simulink model "Copy_of_mpcACCWithSensorFusion"  (R2023b)
settings: Solver=FixedStepAuto  StartTime=0.0  StopTime=34  FixedStep=0.1  RelTol=1e-3
values from neighbouring files (symbols this model uses):
  pfcsubsystem_data =     [pfc_controller_data.mat]    (also in pfc_data.mat; pfc_subsystem_data.mat)
  posSelector = [1,0,0,0,0,0; 0,0,1,0,0,0]    [setUpACCWorkspaceVars.m]
  Ts = 0.1    [mainACCcode.m]    (also in setUpACCWorkspaceVars.m)
undefined symbols (not defined in the file or in its folder): hasLag, InitialLongVel, NumEgoStates, PredictionHorizon
libraries: mpcsigdimcheck_private x19, simulink x2, mpclib x2, trackingutilitieslib x1, drivinglib x1
(part 1 of 2)
settings Model: Creator=The MathWorks, Inc.  LastModifiedBy=Subhadeep Das
settings SolverCC: AlgebraicLoopSolver=TrustRegion  MinimalZcImpactIntegration=on
settings DataIOCC: SaveOutput=off  SignalLogging=off  SaveTime=off  ReturnWorkspaceOutputs=off
settings OptimizationCC: DefaultParameterBehavior=Inlined  InlineInvariantSignals=on  PassReuseOutputArgsAs=Individual arguments  ZeroExternalMemoryAtStartup=off  ZeroInternalMemoryAtStartup=off  OptimizeBlockOrder=speed  EfficientTunableParamExpr=on
settings DebuggingCC: ParameterTunabilityLossMsg=error  UnconnectedInputMsg=warning  UnconnectedOutputMsg=warning  UnconnectedLineMsg=warning  ArithmeticOperatorsInVariantConditions=warning
settings HardwareCC: ProdLongLongMode=on
settings ModelReferenceCC: EnableRefExpFcnMdlSchedulingChecks=on  PropagateVarSize=Only when enabling
settings SFSimCC: SimUseLocalCustomCode=off  MATLABDynamicMemAlloc=off  CustomCodeUndefinedFunction=UseInterfaceOnly  SimTargetLang=C++
settings RTWCC: Description=Embedded Coder  SystemTargetFile=ert.tlc  TemplateMakefile=ert_default_tmf  GenerateReport=on  RTWUseLocalCustomCode=off  BuildConfiguration=Faster Runs  IncludeHyperlinkInReport=on  LaunchReport=on  TargetLang=C++  GenerateTraceInfo=on  GenerateTraceReport=on  GenerateTraceReportSl=on  GenerateTraceReportSf=on  GenerateTraceReportEml=on  GenerateCodeMetricsReport=on  DLArmComputeVersion=19.05
settings CodeAppCC: ForceParamTrailComments=on  IgnoreCustomStorageClasses=off  MaxIdLength=63  OperatorAnnotations=on  SimulinkDataObjDesc=on  SFDataObjDesc=on  CustomSymbolStrFcn=$N$M$F  InsertBlockDesc=on
settings ERTTargetCC: TargetLangStandard=C++03 (ISO)  GenerateSampleERTMain=on  CombineSignalStateStructs=on  SuppressErrorStatus=on  CodeInterfacePackaging=C++ class  InlinedParameterPlacement=NonHierarchical  RootIOFormat=Structure reference  RTWCAPISignals=on  ERTCustomFileTemplate=example_file_process.tlc

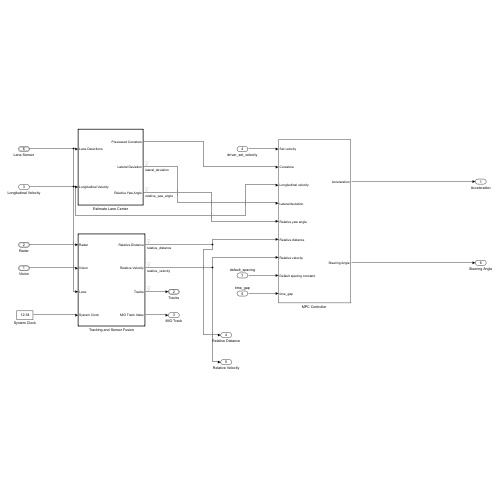
[thumbnail: Simulink's stored preview of the top-level diagram]
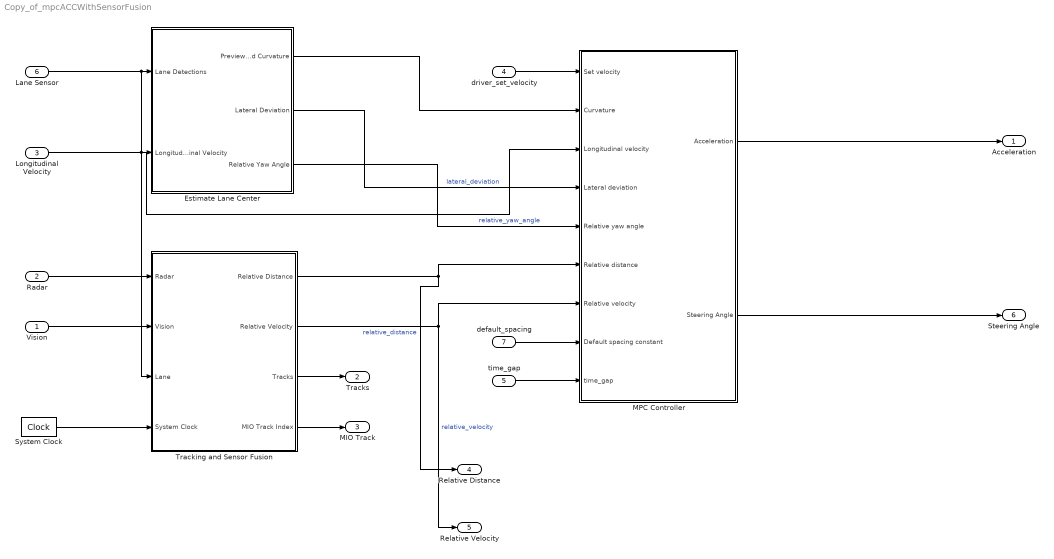
== system Copy_of_mpcACCWithSensorFusion ==
  Vision : Inport  OutDataTypeStr=Bus: BusVision  PortDimensions=[1 1]  SampleTime=[0.10000000000000001,0]  BusOutputAsStruct=on
  Radar : Inport  Port=2  OutDataTypeStr=Bus: BusRadar  PortDimensions=[1 1]  SampleTime=[0.10000000000000001,0]  BusOutputAsStruct=on
  Longitudinal Velocity : Inport  Port=3  OutDataTypeStr=double  PortDimensions=1  SampleTime=[0.10000000000000001,0]
  driver_set_velocity : Inport  Port=4
  time_gap : Inport  Port=5
  Lane Sensor : Inport  Port=6  OutDataTypeStr=Bus: LaneSensor
  default_spacing : Inport  Port=7
  Estimate Lane Center : Subsystem  TreatAsAtomicUnit=on  VariantControl=v2
      settings: RTWFileNameOpts=Use function name
  "MPC Controller " : Subsystem
  System Clock : DigitalClock  SampleTime=Ts
  Tracking and Sensor Fusion : Subsystem  TreatAsAtomicUnit=on
      settings: RTWFileNameOpts=Use function name
  "Acceleration " : Outport  OutDataTypeStr=double  PortDimensions=1  SampleTime=[0.10000000000000001,0]  VectorParamsAs1DForOutWhenUnconnected=off
  Tracks : Outport  Port=2  OutDataTypeStr=Bus:BusMultiObjectTracker1  PortDimensions=[1 1]  SampleTime=[0.10000000000000001,0]  VectorParamsAs1DForOutWhenUnconnected=off  BusOutputAsStruct=on
  MIO Track : Outport  Port=3  OutDataTypeStr=double  PortDimensions=1  SampleTime=[0.10000000000000001,0]  VectorParamsAs1DForOutWhenUnconnected=off  BusOutputAsStruct=on
  Relative Distance : Outport  Port=4
  Relative Velocity : Outport  Port=5
  Steering Angle : Outport  Port=6
  wires:
  Tracking and Sensor Fusion/3(Tracks) -> Tracks/1
  Vision/1 -> Tracking and Sensor Fusion/2(Vision)
  Radar/1 -> Tracking and Sensor Fusion/1(Radar)
  Tracking and Sensor Fusion/4(MIO Track Index) -> MIO Track/1
  Longitudinal Velocity/1 -> "MPC Controller "/3(Longitudinal velocity), Estimate Lane Center/2(Longitudinal Velocity)
  Lane Sensor/1 -> Tracking and Sensor Fusion/3(Lane), Estimate Lane Center/1(Lane Detections)
  System Clock/1 -> Tracking and Sensor Fusion/4(System Clock)
  Tracking and Sensor Fusion/1(Relative Distance) -> Relative Distance/1, "MPC Controller "/6(Relative distance)  "relative_distance"
  Tracking and Sensor Fusion/2(Relative Velocity) -> Relative Velocity/1, "MPC Controller "/7(Relative velocity)  "relative_velocity"
  driver_set_velocity/1 -> "MPC Controller "/1(Set velocity)
  time_gap/1 -> "MPC Controller "/9(time_gap)
  Estimate Lane Center/3(Relative Yaw Angle) -> "MPC Controller "/5(Relative yaw angle)  "relative_yaw_angle"
  Estimate Lane Center/2(Lateral Deviation) -> "MPC Controller "/4(Lateral deviation)  "lateral_deviation"
  Estimate Lane Center/1(Previewed Curvature) -> "MPC Controller "/2(Curvature)
  default_spacing/1 -> "MPC Controller "/8(Default spacing constant)
  "MPC Controller "/1(Acceleration) -> "Acceleration "/1
  "MPC Controller "/2(Steering Angle) -> Steering Angle/1

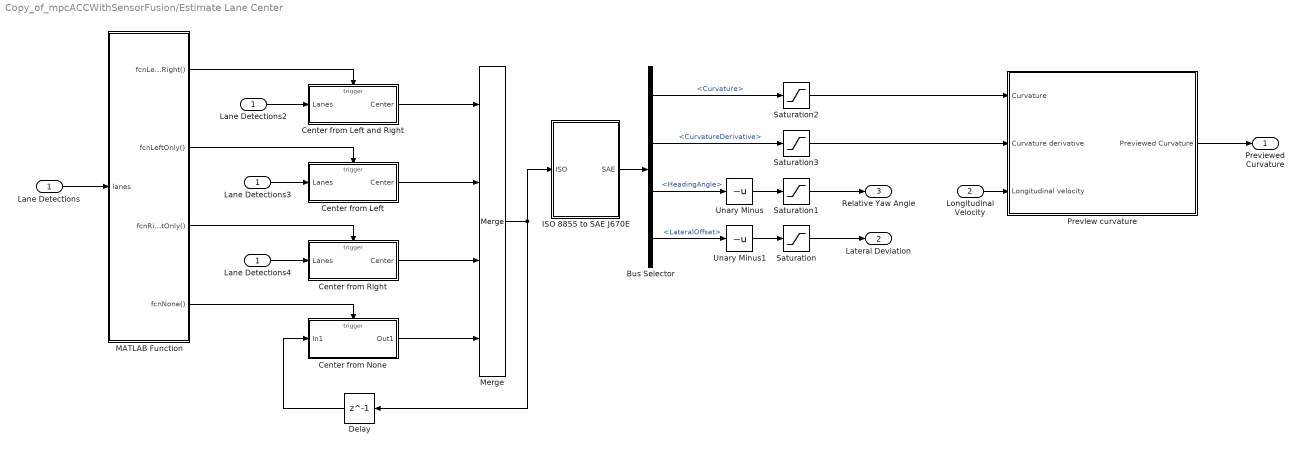
== system Copy_of_mpcACCWithSensorFusion/Estimate Lane Center ==
  Lane Detections : Inport
  Longitudinal Velocity : Inport  Port=2
  Bus Selector : BusSelector  OutputSignals=Curvature,CurvatureDerivative,HeadingAngle,LateralOffset
  Center from Left : Subsystem  TreatAsAtomicUnit=on
  Center from Left and Right : Subsystem  TreatAsAtomicUnit=on
  Center from None : Subsystem  TreatAsAtomicUnit=on
  Center from Right : Subsystem  TreatAsAtomicUnit=on
  Delay : Delay  DelayLength=1
  ISO 8855 to SAE J670E : Subsystem
  Lane Detections2 : InportShadow
  Lane Detections3 : InportShadow
  Lane Detections4 : InportShadow
  MATLAB Function : MATLAB Function  TreatAsAtomicUnit=on
  Merge : Merge  Inputs=4
  Preview curvature : Subsystem
  Saturation : Saturate
  Saturation1 : Saturate  UpperLimit=0.6  LowerLimit=-0.6
  Saturation2 : Saturate  UpperLimit=0.15  LowerLimit=-0.15
  Saturation3 : Saturate  UpperLimit=0.06  LowerLimit=-0.06
  Unary Minus : UnaryMinus
  Unary Minus1 : UnaryMinus
  Previewed Curvature : Outport  VectorParamsAs1DForOutWhenUnconnected=off
  Lateral Deviation : Outport  Port=2  VectorParamsAs1DForOutWhenUnconnected=off
  Relative Yaw Angle : Outport  Port=3  VectorParamsAs1DForOutWhenUnconnected=off
  wires:
  Center from Right/1(Center) -> Merge/3
  Lane Detections3/1 -> Center from Left/1(Lanes)
  Lane Detections4/1 -> Center from Right/1(Lanes)
  MATLAB Function/2(fcnLeftOnly()) -> Center from Left/Trigger
  Center from None/1(Out1) -> Merge/4
  MATLAB Function/1(fcnLeftAndRight()) -> Center from Left and Right/Trigger
  Delay/1 -> Center from None/1(In1)
  Center from Left and Right/1(Center) -> Merge/1
  Lane Detections/1 -> MATLAB Function/1(lanes)
  Lane Detections2/1 -> Center from Left and Right/1(Lanes)
  MATLAB Function/3(fcnRightOnly()) -> Center from Right/Trigger
  MATLAB Function/4(fcnNone()) -> Center from None/Trigger
  Center from Left/1(Center) -> Merge/2
  Merge/1 -> ISO 8855 to SAE J670E/1(ISO), Delay/1
  Saturation3/1 -> Preview curvature/2(Curvature derivative)
  Saturation2/1 -> Preview curvature/1(Curvature)
  Saturation1/1 -> Relative Yaw Angle/1
  Saturation/1 -> Lateral Deviation/1
  Unary Minus/1 -> Saturation1/1
  Preview curvature/1(Previewed Curvature) -> Previewed Curvature/1
  Longitudinal Velocity/1 -> Preview curvature/3(Longitudinal velocity)
  Bus Selector/2 -> Saturation3/1  "<CurvatureDerivative>"
  Bus Selector/1 -> Saturation2/1  "<Curvature>"
  Unary Minus1/1 -> Saturation/1
  Bus Selector/4 -> Unary Minus1/1  "<LateralOffset>"
  Bus Selector/3 -> Unary Minus/1  "<HeadingAngle>"
  ISO 8855 to SAE J670E/1(SAE) -> Bus Selector/1

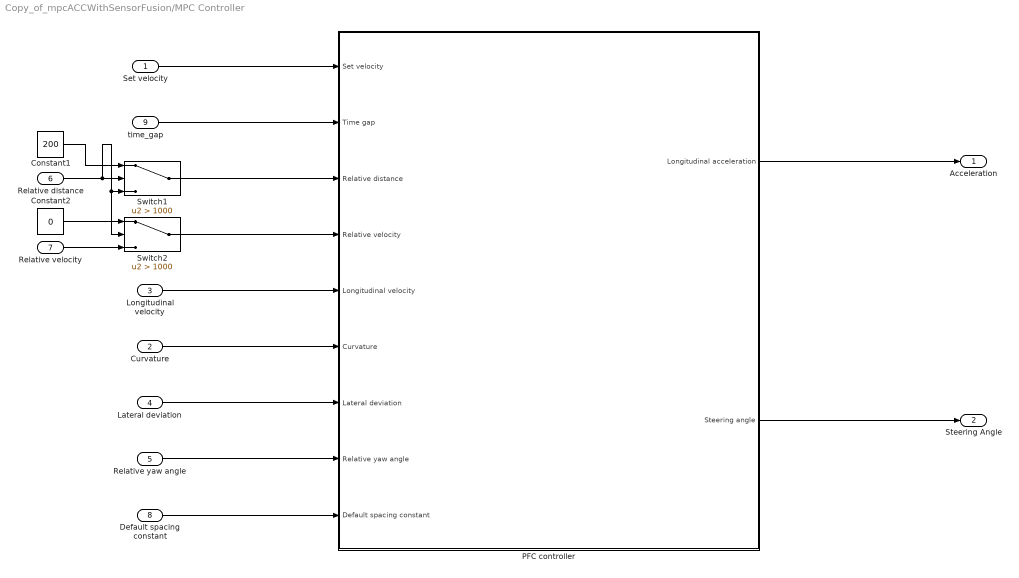
== system Copy_of_mpcACCWithSensorFusion/MPC Controller  ==
  Set velocity : Inport
  Curvature : Inport  Port=2
  Longitudinal velocity : Inport  Port=3
  Lateral deviation : Inport  Port=4
  Relative yaw angle : Inport  Port=5
  Relative distance : Inport  Port=6
  Relative velocity : Inport  Port=7
  Default spacing constant : Inport  Port=8
  time_gap : Inport  Port=9
  Constant1 : Constant  Value=200
  Constant2 : Constant  Value=0
  PFC controller : Subsystem  TreatAsAtomicUnit=on  VariantControl=Variant2
      settings: LibrarySourceBlock=mpcadaslib/Path Following Control System  RTWFileNameOpts=Use function name
  Switch1 : Switch  Criteria=u2 > Threshold  Threshold=1000  SaturateOnIntegerOverflow=off  InputSameDT=off
  Switch2 : Switch  Criteria=u2 > Threshold  Threshold=1000  SaturateOnIntegerOverflow=off  InputSameDT=off
  Acceleration : Outport  VectorParamsAs1DForOutWhenUnconnected=off
  Steering Angle : Outport  Port=2  VectorParamsAs1DForOutWhenUnconnected=off
  wires:
  PFC controller/1(Longitudinal acceleration) -> Acceleration/1
  PFC controller/2(Steering angle) -> Steering Angle/1
  Set velocity/1 -> PFC controller/1(Set velocity)
  time_gap/1 -> PFC controller/2(Time gap)
  Relative distance/1 -> Switch2/2, Switch1/3, Switch1/2
  Constant1/1 -> Switch1/1
  Switch1/1 -> PFC controller/3(Relative distance)
  Relative velocity/1 -> Switch2/3
  Constant2/1 -> Switch2/1
  Switch2/1 -> PFC controller/4(Relative velocity)
  Longitudinal velocity/1 -> PFC controller/5(Longitudinal velocity)
  Curvature/1 -> PFC controller/6(Curvature)
  Lateral deviation/1 -> PFC controller/7(Lateral deviation)
  Relative yaw angle/1 -> PFC controller/8(Relative yaw angle)
  Default spacing constant/1 -> PFC controller/9(Default spacing constant)

== system Copy_of_mpcACCWithSensorFusion/Tracking and Sensor Fusion ==
  note: Sensor Fusion
  Radar : Inport  OutDataTypeStr=Bus: BusRadar  PortDimensions=[1 1]  BusOutputAsStruct=on
  Vision : Inport  Port=2  OutDataTypeStr=Bus: BusVision  PortDimensions=[1 1]  BusOutputAsStruct=on
  Lane : Inport  Port=3  OutDataTypeStr=Bus: LaneSensor  BusOutputAsStruct=on
  System Clock : Inport  Port=4  OutDataTypeStr=double  PortDimensions=[1 1]
  Detection Concatenation1 : trackingutilitieslib/Detection Concatenation  NumInputs=2  BusNameSource=Auto  BusName=BusDetectionConcatenation1  SimulateUsing=Interpreted execution
  Find Lead Car : MATLAB Function  TreatAsAtomicUnit=on
  Multi-Object Tracker : drivinglib/Multi-Object Tracker  TrackerIndex=uint32( 0 )  FilterInitializationFcn=initcvekf  AssignmentThreshold=assigThresh  ConfirmationThreshold=[ 2, 3 ]  DeletionThreshold=[ 5, 5 ]  MaxNumTracks=numTracks  MaxNumSensors=numSensors  OOSMHandling=Terminate  StateParametersSimulink=struct  HasStateParametersInput=off  TimeInputSource=Input port  HasCostMatrixInput=off  HasDetectableTrackIDsInput=off  BusNameSource=Property  BusName=BusMultiObjectTracker1  TentativeTracksOutputPort=off  AllTracksOutputPort=off  SimulateUsing=Interpreted execution
  Position Selector : Constant  Value=posSelector
  Relative Distance : Outport  VectorParamsAs1DForOutWhenUnconnected=off
  Relative Velocity : Outport  Port=2  VectorParamsAs1DForOutWhenUnconnected=off
  Tracks : Outport  Port=3  OutDataTypeStr=Bus:BusMultiObjectTracker1  PortDimensions=[1 1]  VectorParamsAs1DForOutWhenUnconnected=off  BusOutputAsStruct=on
  MIO Track Index : Outport  Port=4  VectorParamsAs1DForOutWhenUnconnected=off
  wires:
  Find Lead Car/2(vx) -> Relative Velocity/1
  Find Lead Car/3(mioTrackIndex) -> MIO Track Index/1
  Find Lead Car/1(x) -> Relative Distance/1
  Position Selector/1 -> Find Lead Car/3(positionSelector)
  Lane/1 -> Find Lead Car/2(lane)
  Detection Concatenation1/1 -> Multi-Object Tracker/1
  Multi-Object Tracker/1 -> Find Lead Car/1(confirmedTracks), Tracks/1
  System Clock/1 -> Multi-Object Tracker/2
  Vision/1 -> Detection Concatenation1/1
  Radar/1 -> Detection Concatenation1/2

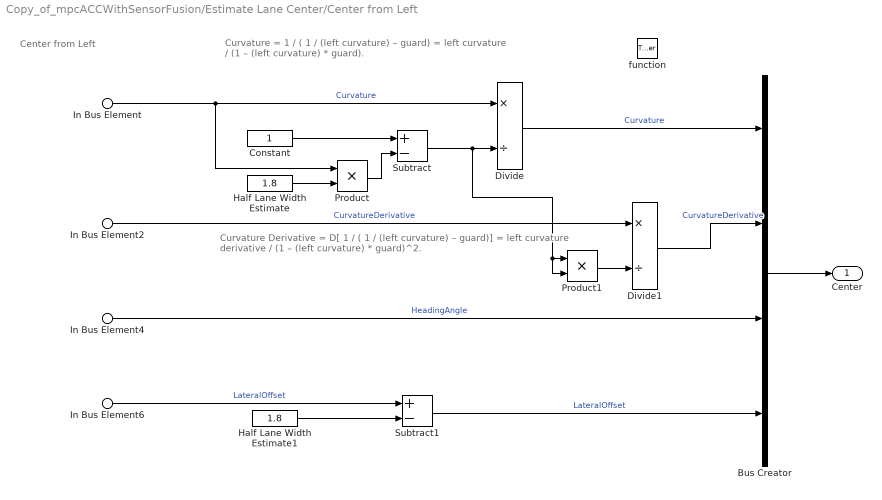
== system Copy_of_mpcACCWithSensorFusion/Estimate Lane Center/Center from Left ==
  note: Curvature Derivative
      | = D[ 1 / ( 1 / (left curvature) – guard)]
      | = left curvature derivative / (1 – (left curvature) * guard)^2.
  note: Center from Left
  note: Curvature
      | = 1 / ( 1 / (left curvature) – guard)
      | = left curvature / (1 – (left curvature) * guard).
  In Bus Element : Inport  PortName=Lanes  Element=Left.Curvature
  In Bus Element2 : Inport  PortName=Lanes  Element=Left.CurvatureDerivative
  In Bus Element4 : Inport  PortName=Lanes  Element=Left.HeadingAngle
  In Bus Element6 : Inport  PortName=Lanes  Element=Left.LateralOffset
  function : TriggerPort  TriggerType=function-call  VariantControl=Variant
  Bus Creator : BusCreator  Inputs=4
  Constant : Constant  OutDataTypeStr=Inherit: Inherit via back propagation
  Divide : Product  Inputs=*/
  Divide1 : Product  Inputs=*/
  Half Lane Width Estimate : Constant  Value=1.8  OutDataTypeStr=Inherit: Inherit via back propagation
  Half Lane Width Estimate1 : Constant  Value=1.8  OutDataTypeStr=Inherit: Inherit via back propagation
  Product : Product
  Product1 : Product
  Subtract : Sum  Inputs=+-
  Subtract1 : Sum  Inputs=+-
  Center : Outport  VectorParamsAs1DForOutWhenUnconnected=off
  wires:
  Product/1 -> Subtract/2
  Half Lane Width Estimate1/1 -> Subtract1/2
  In Bus Element6/1 -> Subtract1/1  "LateralOffset"
  Product1/1 -> Divide1/2
  In Bus Element2/1 -> Divide1/1  "CurvatureDerivative"
  Constant/1 -> Subtract/1
  Half Lane Width Estimate/1 -> Product/2
  Subtract/1 -> Divide/2, Product1/1, Product1/2
  In Bus Element/1 -> Divide/1, Product/1  "Curvature"
  Subtract1/1 -> Bus Creator/4  "LateralOffset"
  In Bus Element4/1 -> Bus Creator/3  "HeadingAngle"
  Divide/1 -> Bus Creator/1  "Curvature"
  Divide1/1 -> Bus Creator/2  "CurvatureDerivative"
  Bus Creator/1 -> Center/1

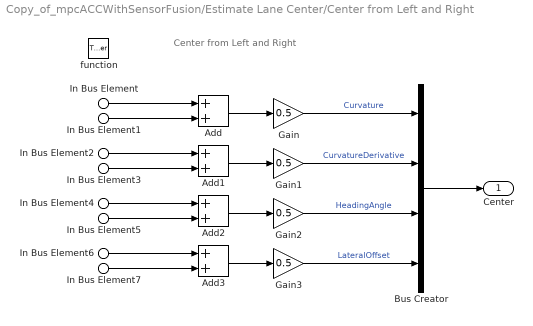
== system Copy_of_mpcACCWithSensorFusion/Estimate Lane Center/Center from Left and Right ==
  note: Center from Left and Right
  In Bus Element : Inport  PortName=Lanes  Element=Left.Curvature
  In Bus Element2 : Inport  PortName=Lanes  Element=Left.CurvatureDerivative
  In Bus Element4 : Inport  PortName=Lanes  Element=Left.HeadingAngle
  In Bus Element6 : Inport  PortName=Lanes  Element=Left.LateralOffset
  In Bus Element1 : Inport  PortName=Lanes  Element=Right.Curvature
  In Bus Element3 : Inport  PortName=Lanes  Element=Right.CurvatureDerivative
  In Bus Element5 : Inport  PortName=Lanes  Element=Right.HeadingAngle
  In Bus Element7 : Inport  PortName=Lanes  Element=Right.LateralOffset
  function : TriggerPort  TriggerType=function-call  VariantControl=Variant
  Add{,1..3} (4 alike) : Sum
  Bus Creator : BusCreator  Inputs=4
  Gain{,1..3} (4 alike) : Gain  Gain=0.5
  Center : Outport  VectorParamsAs1DForOutWhenUnconnected=off
  wires:
  In Bus Element6/1 -> Add3/1
  In Bus Element7/1 -> Add3/2
  In Bus Element5/1 -> Add2/2
  In Bus Element4/1 -> Add2/1
  In Bus Element3/1 -> Add1/2
  In Bus Element2/1 -> Add1/1
  In Bus Element1/1 -> Add/2
  In Bus Element/1 -> Add/1
  Bus Creator/1 -> Center/1
  Gain3/1 -> Bus Creator/4  "LateralOffset"
  Add3/1 -> Gain3/1
  Gain2/1 -> Bus Creator/3  "HeadingAngle"
  Add2/1 -> Gain2/1
  Gain1/1 -> Bus Creator/2  "CurvatureDerivative"
  Add1/1 -> Gain1/1
  Gain/1 -> Bus Creator/1  "Curvature"
  Add/1 -> Gain/1

== system Copy_of_mpcACCWithSensorFusion/Estimate Lane Center/Center from None ==
  In1 : Inport
  function : TriggerPort  TriggerType=function-call  VariantControl=Variant
  Out1 : Outport  VectorParamsAs1DForOutWhenUnconnected=off
  wires:
  In1/1 -> Out1/1

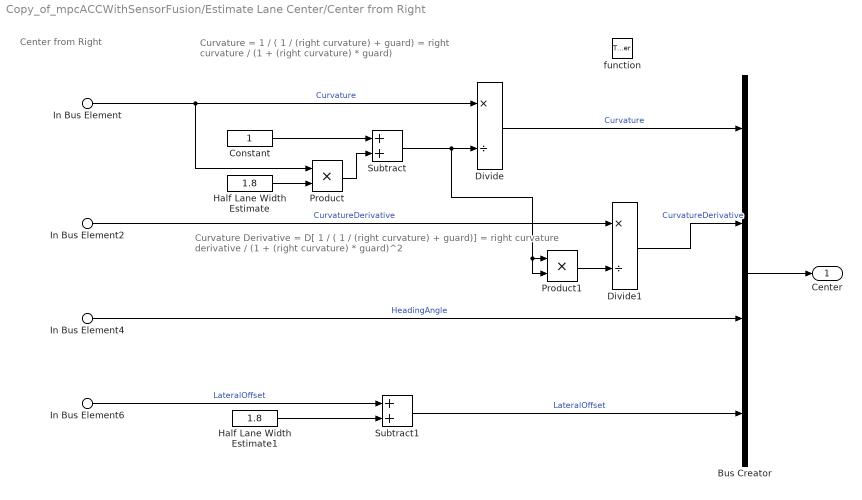
== system Copy_of_mpcACCWithSensorFusion/Estimate Lane Center/Center from Right ==
  note: Curvature Derivative
      | = D[ 1 / ( 1 / (right curvature) + guard)]
      | = right curvature derivative / (1 + (right curvature) * guard)^2
  note: Curvature
      | = 1 / ( 1 / (right curvature) + guard)
      | = right curvature / (1 + (right curvature) * guard)
  note: Center from Right
  In Bus Element : Inport  PortName=Lanes  Element=Right.Curvature
  In Bus Element2 : Inport  PortName=Lanes  Element=Right.CurvatureDerivative
  In Bus Element4 : Inport  PortName=Lanes  Element=Right.HeadingAngle
  In Bus Element6 : Inport  PortName=Lanes  Element=Right.LateralOffset
  function : TriggerPort  TriggerType=function-call  VariantControl=Variant
  Bus Creator : BusCreator  Inputs=4
  Constant : Constant  OutDataTypeStr=Inherit: Inherit via back propagation
  Divide : Product  Inputs=*/
  Divide1 : Product  Inputs=*/
  Half Lane Width Estimate : Constant  Value=1.8  OutDataTypeStr=Inherit: Inherit via back propagation
  Half Lane Width Estimate1 : Constant  Value=1.8  OutDataTypeStr=Inherit: Inherit via back propagation
  Product : Product
  Product1 : Product
  Subtract : Sum
  Subtract1 : Sum
  Center : Outport  VectorParamsAs1DForOutWhenUnconnected=off
  wires:
  Half Lane Width Estimate/1 -> Product/2
  Product/1 -> Subtract/2
  Constant/1 -> Subtract/1
  Subtract/1 -> Divide/2, Product1/1, Product1/2
  In Bus Element/1 -> Divide/1, Product/1  "Curvature"
  Bus Creator/1 -> Center/1
  Subtract1/1 -> Bus Creator/4  "LateralOffset"
  Divide/1 -> Bus Creator/1  "Curvature"
  In Bus Element6/1 -> Subtract1/1  "LateralOffset"
  Half Lane Width Estimate1/1 -> Subtract1/2
  In Bus Element4/1 -> Bus Creator/3  "HeadingAngle"
  Product1/1 -> Divide1/2
  Divide1/1 -> Bus Creator/2  "CurvatureDerivative"
  In Bus Element2/1 -> Divide1/1  "CurvatureDerivative"

== system Copy_of_mpcACCWithSensorFusion/Estimate Lane Center/ISO 8855 to SAE J670E ==
  ISO : Inport
  Bus Creator : BusCreator  Inputs=4
  Bus Selector : BusSelector  OutputSignals=CurvatureDerivative,Curvature,HeadingAngle,LateralOffset
  Signal Specification : SignalSpecification  Unit=1/m^2
  Signal Specification1 : SignalSpecification  Unit=1/m
  Signal Specification2 : SignalSpecification  Unit=rad
  Signal Specification3 : SignalSpecification  Unit=m
  Unary Minus{,1..3} (4 alike) : UnaryMinus
  SAE : Outport  VectorParamsAs1DForOutWhenUnconnected=off
  wires:
  ISO/1 -> Bus Selector/1
  Bus Selector/2 -> Unary Minus/1  "<Curvature>"
  Bus Selector/1 -> Unary Minus1/1  "<CurvatureDerivative>"
  Bus Selector/3 -> Unary Minus2/1  "<HeadingAngle>"
  Bus Selector/4 -> Unary Minus3/1  "<LateralOffset>"
  Bus Creator/1 -> SAE/1
  Signal Specification/1 -> Bus Creator/2  "Curvature"
  Unary Minus1/1 -> Signal Specification1/1
  Unary Minus2/1 -> Signal Specification2/1
  Unary Minus3/1 -> Signal Specification3/1
  Unary Minus/1 -> Signal Specification/1
  Signal Specification1/1 -> Bus Creator/1  "CurvatureDerivative"
  Signal Specification2/1 -> Bus Creator/3  "HeadingAngle"
  Signal Specification3/1 -> Bus Creator/4  "LateralOffset"

== system Copy_of_mpcACCWithSensorFusion/Estimate Lane Center/Preview curvature ==
  Curvature : Inport
  Curvature derivative : Inport  Port=2
  Longitudinal velocity : Inport  Port=3
  Gain : Gain  Gain=[0:Ts:PredictionHorizon*Ts]'
  Product : Product
  Sum : Sum
  Previewed Curvature : Outport  VectorParamsAs1DForOutWhenUnconnected=off
  wires:
  Sum/1 -> Previewed Curvature/1
  Curvature/1 -> Sum/1
  Gain/1 -> Sum/2
  Product/1 -> Gain/1
  Longitudinal velocity/1 -> Product/2
  Curvature derivative/1 -> Product/1

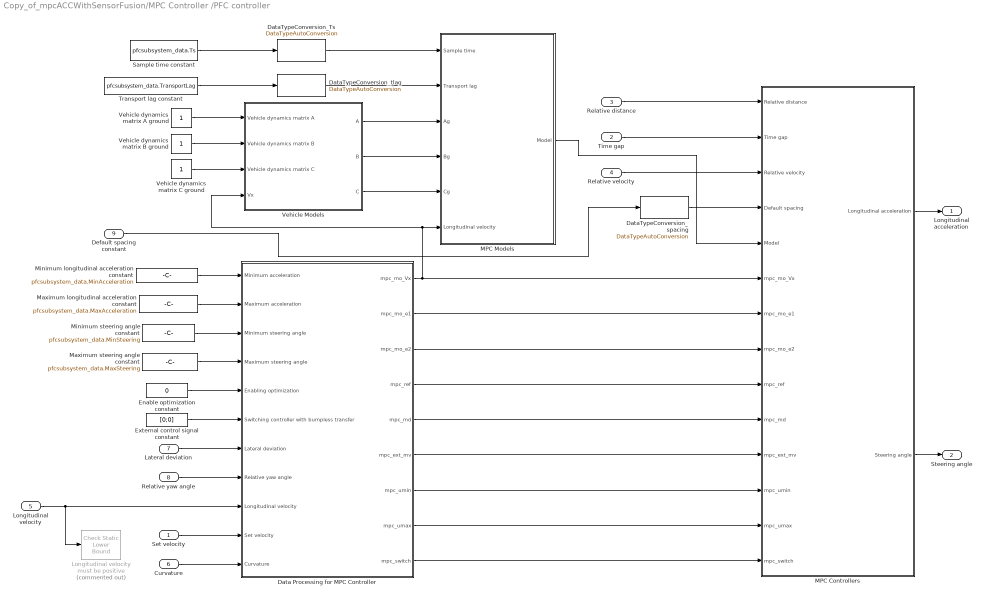
== system Copy_of_mpcACCWithSensorFusion/MPC Controller /PFC controller ==
  Set velocity : Inport
  Time gap : Inport  Port=2
  Relative distance : Inport  Port=3
  Relative velocity : Inport  Port=4
  Longitudinal velocity : Inport  Port=5
  Curvature : Inport  Port=6
  Lateral deviation : Inport  Port=7
  Relative yaw angle : Inport  Port=8
  Default spacing constant : Inport  Port=9
  Data Processing for MPC Controller : Subsystem
  DataTypeConversion_Ts : mpcsigdimcheck_private/DataTypeAutoConversion  datatypestr=pfcsubsystem_data.DataType
  DataTypeConversion_spacing : mpcsigdimcheck_private/DataTypeAutoConversion  datatypestr=pfcsubsystem_data.DataType
  DataTypeConversion_tlag : mpcsigdimcheck_private/DataTypeAutoConversion  datatypestr=pfcsubsystem_data.DataType
  Enable optimization constant : Constant  Value=0  OutDataTypeStr=pfcsubsystem_data.DataType
  External control signal constant : Constant  Value=[0;0]  VectorParams1D=off  OutDataTypeStr=pfcsubsystem_data.DataType
  Longitudinal velocity must be positive : simulink/Model Verification/Check Static  Lower Bound  Description=0 < u  Commented=on  min=0  min_included=off  enabled=on  stopWhenAssertionFail=on  export=off  icon=graphic
  MPC Controllers : Subsystem  Variant=on  VariantControlMode=label  VariantControl=Variant1  LabelModeActiveChoice=pathFollowingHasSpacingCtrl
  MPC Models : Subsystem  Variant=on  VariantControlMode=label  VariantControl=Variant1  LabelModeActiveChoice=pathFollowingHasSpacingCtrl
  Maximum longitudinal acceleration constant : Constant  Value=pfcsubsystem_data.MaxAcceleration  OutDataTypeStr=pfcsubsystem_data.DataType
  Maximum steering angle constant : Constant  Value=pfcsubsystem_data.MaxSteering  OutDataTypeStr=pfcsubsystem_data.DataType
  Minimum longitudinal acceleration constant : Constant  Value=pfcsubsystem_data.MinAcceleration  OutDataTypeStr=pfcsubsystem_data.DataType
  Minimum steering angle constant : Constant  Value=pfcsubsystem_data.MinSteering  OutDataTypeStr=pfcsubsystem_data.DataType
  Sample time constant : Constant  Value=pfcsubsystem_data.Ts  OutDataTypeStr=pfcsubsystem_data.DataType
  Transport lag constant : Constant  Value=pfcsubsystem_data.TransportLag  OutDataTypeStr=pfcsubsystem_data.DataType
  Vehicle Models : Subsystem  Variant=on  VariantControlMode=label  VariantControl=Variant1  LabelModeActiveChoice=useVehicleParameters
  Vehicle dynamics matrix A ground : Constant  OutDataTypeStr=pfcsubsystem_data.DataType
  Vehicle dynamics matrix B ground : Constant  OutDataTypeStr=pfcsubsystem_data.DataType
  Vehicle dynamics matrix C ground : Constant  OutDataTypeStr=pfcsubsystem_data.DataType
  Longitudinal acceleration : Outport  PortDimensions=1  VectorParamsAs1DForOutWhenUnconnected=off
  Steering angle : Outport  Port=2  VectorParamsAs1DForOutWhenUnconnected=off
  wires:
  MPC Controllers/1(" Longitudinal acceleration") -> Longitudinal acceleration/1
  Default spacing constant/1 -> DataTypeConversion_spacing/1
  Data Processing for MPC Controller/9(mpc_switch) -> MPC Controllers/14("mpc_switch ")
  MPC Models/1(" Model") -> MPC Controllers/5("Model ")
  Data Processing for MPC Controller/8(mpc_umax) -> MPC Controllers/13("mpc_umax ")
  MPC Controllers/2("  Steering angle") -> Steering angle/1
  Data Processing for MPC Controller/1(mpc_mo_Vx) -> MPC Models/6("Longitudinal velocity "), Vehicle Models/4("Vx "), MPC Controllers/6("mpc_mo_Vx ")
  Data Processing for MPC Controller/5(mpc_md) -> MPC Controllers/10("mpc_md ")
  Data Processing for MPC Controller/3(mpc_mo_e2) -> MPC Controllers/8("mpc_mo_e2 ")
  Data Processing for MPC Controller/4(mpc_ref) -> MPC Controllers/9("mpc_ref ")
  Longitudinal velocity/1 -> Longitudinal velocity must be positive/1, Data Processing for MPC Controller/9(Longitudinal velocity)
  Data Processing for MPC Controller/2(mpc_mo_e1) -> MPC Controllers/7("mpc_mo_e1 ")
  Data Processing for MPC Controller/6(mpc_ext_mv) -> MPC Controllers/11("mpc_ext_mv ")
  Data Processing for MPC Controller/7(mpc_umin) -> MPC Controllers/12("mpc_umin ")
  Curvature/1 -> Data Processing for MPC Controller/11(Curvature)
  Set velocity/1 -> Data Processing for MPC Controller/10(Set velocity)
  Lateral deviation/1 -> Data Processing for MPC Controller/7(Lateral deviation)
  Relative yaw angle/1 -> Data Processing for MPC Controller/8(Relative yaw angle)
  Maximum longitudinal acceleration constant/1 -> Data Processing for MPC Controller/2(Maximum acceleration)
  Maximum steering angle constant/1 -> Data Processing for MPC Controller/4(Maximum steering angle)
  Enable optimization constant/1 -> Data Processing for MPC Controller/5(Enabling optimization)
  External control signal constant/1 -> Data Processing for MPC Controller/6(Switching controller with bumpless transfer)
  Minimum longitudinal acceleration constant/1 -> Data Processing for MPC Controller/1(Minimum acceleration)
  Minimum steering angle constant/1 -> Data Processing for MPC Controller/3(Minimum steering angle)
  Vehicle Models/1(" A") -> MPC Models/3(Ag)
  Vehicle Models/2(" B") -> MPC Models/4(Bg)
  Vehicle Models/3(" C") -> MPC Models/5(Cg)
  Transport lag constant/1 -> DataTypeConversion_tlag/1
  Sample time constant/1 -> DataTypeConversion_Ts/1
  Time gap/1 -> MPC Controllers/2("Time gap ")
  Relative distance/1 -> MPC Controllers/1("Relative distance ")
  Relative velocity/1 -> MPC Controllers/3("Relative velocity ")
  Vehicle dynamics matrix A ground/1 -> Vehicle Models/1(Vehicle dynamics matrix A)
  Vehicle dynamics matrix C ground/1 -> Vehicle Models/3(Vehicle dynamics matrix C)
  Vehicle dynamics matrix B ground/1 -> Vehicle Models/2(Vehicle dynamics matrix B)
  DataTypeConversion_Ts/1 -> MPC Models/1(Sample time)
  DataTypeConversion_tlag/1 -> MPC Models/2(Transport lag)
  DataTypeConversion_spacing/1 -> MPC Controllers/4("Default spacing ")

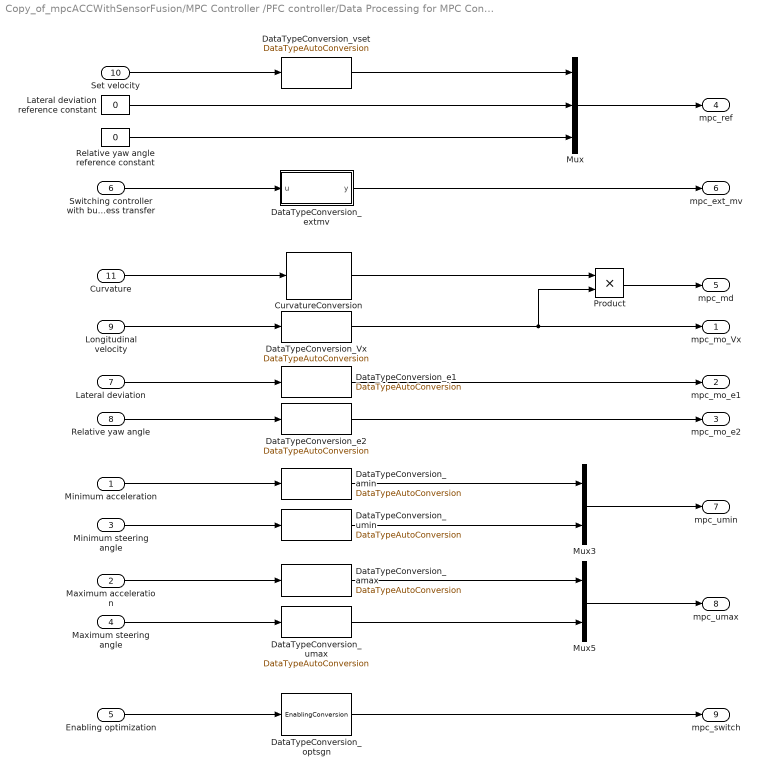
== system Copy_of_mpcACCWithSensorFusion/MPC Controller /PFC controller/Data Processing for MPC Controller ==
  Minimum acceleration : Inport
  Maximum acceleration : Inport  Port=2
  Minimum steering angle : Inport  Port=3
  Maximum steering angle : Inport  Port=4
  Enabling optimization : Inport  Port=5
  Switching controller with bumpless transfer : Inport  Port=6
  Lateral deviation : Inport  Port=7
  Relative yaw angle : Inport  Port=8
  Longitudinal velocity : Inport  Port=9
  Set velocity : Inport  Port=10
  Curvature : Inport  Port=11
  CurvatureConversion : mpcsigdimcheck_private/CurvatureConversion  datatypestr=pfcsubsystem_data.DataType  p=pfcsubsystem_data.Controller.PredictionHorizon
  DataTypeConversion_Vx : mpcsigdimcheck_private/DataTypeAutoConversion  datatypestr=pfcsubsystem_data.DataType
  DataTypeConversion_amax : mpcsigdimcheck_private/DataTypeAutoConversion  datatypestr=pfcsubsystem_data.DataType
  DataTypeConversion_amin : mpcsigdimcheck_private/DataTypeAutoConversion  datatypestr=pfcsubsystem_data.DataType
  DataTypeConversion_e1 : mpcsigdimcheck_private/DataTypeAutoConversion  datatypestr=pfcsubsystem_data.DataType
  DataTypeConversion_e2 : mpcsigdimcheck_private/DataTypeAutoConversion  datatypestr=pfcsubsystem_data.DataType
  DataTypeConversion_extmv : MATLAB Function  TreatAsAtomicUnit=on  mask(MPCDataTypeAutoConversion){datatypestr=pfcsubsystem_data.DataType}
      mask prompts: datatypestr "Data type"
      mask init:
      | isDouble = strcmp(datatypestr,'double');
  DataTypeConversion_optsgn : mpcsigdimcheck_private/EnablingConversion  SystemSampleTime=-1  VariantActivationTime=update diagram  AllowFlexibleInterface=on  Latency=0  AutoFrameSizeCalculation=off
  DataTypeConversion_umax : mpcsigdimcheck_private/DataTypeAutoConversion  datatypestr=pfcsubsystem_data.DataType
  DataTypeConversion_umin : mpcsigdimcheck_private/DataTypeAutoConversion  datatypestr=pfcsubsystem_data.DataType
  DataTypeConversion_vset : mpcsigdimcheck_private/DataTypeAutoConversion  datatypestr=pfcsubsystem_data.DataType
  Lateral deviation reference constant : Constant  Value=0  OutDataTypeStr=pfcsubsystem_data.DataType
  Mux : Mux  Inputs=3
  Mux3 : Mux  Inputs=2
  Mux5 : Mux  Inputs=2
  Product : Product
  "Relative yaw angle reference constant " : Constant  Value=0  OutDataTypeStr=pfcsubsystem_data.DataType
  mpc_mo_Vx : Outport  VectorParamsAs1DForOutWhenUnconnected=off
  mpc_mo_e1 : Outport  Port=2  VectorParamsAs1DForOutWhenUnconnected=off
  mpc_mo_e2 : Outport  Port=3  VectorParamsAs1DForOutWhenUnconnected=off
  mpc_ref : Outport  Port=4  VectorParamsAs1DForOutWhenUnconnected=off
  mpc_md : Outport  Port=5  VectorParamsAs1DForOutWhenUnconnected=off
  mpc_ext_mv : Outport  Port=6  VectorParamsAs1DForOutWhenUnconnected=off
  mpc_umin : Outport  Port=7  VectorParamsAs1DForOutWhenUnconnected=off
  mpc_umax : Outport  Port=8  VectorParamsAs1DForOutWhenUnconnected=off
  mpc_switch : Outport  Port=9  VectorParamsAs1DForOutWhenUnconnected=off
  wires:
  Longitudinal velocity/1 -> DataTypeConversion_Vx/1
  Curvature/1 -> CurvatureConversion/1
  Mux5/1 -> mpc_umax/1
  Lateral deviation reference constant/1 -> Mux/2
  Maximum steering angle/1 -> DataTypeConversion_umax/1
  Minimum steering angle/1 -> DataTypeConversion_umin/1
  DataTypeConversion_amin/1 -> Mux3/1
  CurvatureConversion/1 -> Product/1
  Product/1 -> mpc_md/1
  DataTypeConversion_e2/1 -> mpc_mo_e2/1
  Maximum acceleration/1 -> DataTypeConversion_amax/1
  Lateral deviation/1 -> DataTypeConversion_e1/1
  DataTypeConversion_umin/1 -> Mux3/2
  DataTypeConversion_amax/1 -> Mux5/1
  DataTypeConversion_Vx/1 -> mpc_mo_Vx/1, Product/2
  DataTypeConversion_umax/1 -> Mux5/2
  Minimum acceleration/1 -> DataTypeConversion_amin/1
  Set velocity/1 -> DataTypeConversion_vset/1
  Switching controller with bumpless transfer/1 -> DataTypeConversion_extmv/1(u)
  "Relative yaw angle reference constant "/1 -> Mux/3
  DataTypeConversion_extmv/1(y) -> mpc_ext_mv/1
  Mux3/1 -> mpc_umin/1
  Relative yaw angle/1 -> DataTypeConversion_e2/1
  DataTypeConversion_vset/1 -> Mux/1
  Mux/1 -> mpc_ref/1
  DataTypeConversion_e1/1 -> mpc_mo_e1/1
  Enabling optimization/1 -> DataTypeConversion_optsgn/1
  DataTypeConversion_optsgn/1 -> mpc_switch/1

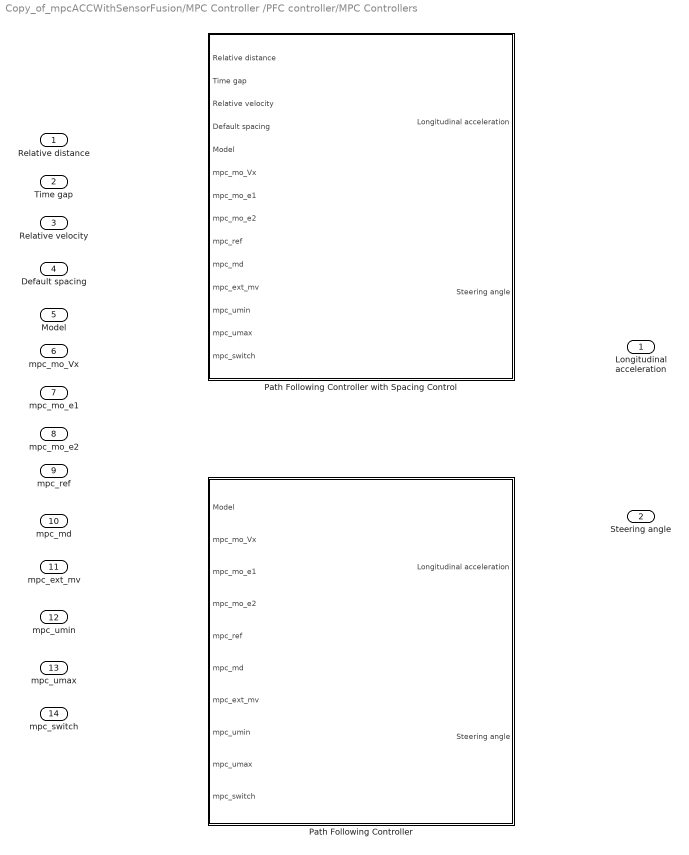
== system Copy_of_mpcACCWithSensorFusion/MPC Controller /PFC controller/MPC Controllers ==
  "Relative distance " : Inport
  "Time gap " : Inport  Port=2
  "Relative velocity " : Inport  Port=3
  "Default spacing " : Inport  Port=4
  "Model " : Inport  Port=5
  "mpc_mo_Vx " : Inport  Port=6
  "mpc_mo_e1 " : Inport  Port=7
  "mpc_mo_e2 " : Inport  Port=8
  "mpc_ref " : Inport  Port=9
  "mpc_md " : Inport  Port=10
  "mpc_ext_mv " : Inport  Port=11
  "mpc_umin " : Inport  Port=12
  "mpc_umax " : Inport  Port=13
  "mpc_switch " : Inport  Port=14
  Path Following Controller : Subsystem  VariantControl=pathFollowingNoSpacingCtrl
  Path Following Controller with Spacing Control : Subsystem  VariantControl=pathFollowingHasSpacingCtrl
  " Longitudinal acceleration" : Outport  VectorParamsAs1DForOutWhenUnconnected=off
  "  Steering angle" : Outport  Port=2  VectorParamsAs1DForOutWhenUnconnected=off

== system Copy_of_mpcACCWithSensorFusion/MPC Controller /PFC controller/MPC Models ==
  Sample time : Inport
  Transport lag : Inport  Port=2
  Ag : Inport  Port=3
  Bg : Inport  Port=4
  Cg : Inport  Port=5
  "Longitudinal velocity " : Inport  Port=6
  MPC Model : Subsystem  VariantControl=pathFollowingNoSpacingCtrl
  MPC Model with Spacing Control : Subsystem  VariantControl=pathFollowingHasSpacingCtrl
  " Model" : Outport  VectorParamsAs1DForOutWhenUnconnected=off

== system Copy_of_mpcACCWithSensorFusion/MPC Controller /PFC controller/Vehicle Models ==
  Vehicle dynamics matrix A : Inport
  Vehicle dynamics matrix B : Inport  Port=2
  Vehicle dynamics matrix C : Inport  Port=3
  "Vx " : Inport  Port=4
  Vehicle external model : Subsystem  VariantControl=useVehicleModel
  Vehicle parametric model : Subsystem  VariantControl=useVehicleParameters
  " A" : Outport  VectorParamsAs1DForOutWhenUnconnected=off
  " B" : Outport  Port=2  VectorParamsAs1DForOutWhenUnconnected=off
  " C" : Outport  Port=3  VectorParamsAs1DForOutWhenUnconnected=off

== system Copy_of_mpcACCWithSensorFusion/MPC Controller /PFC controller/MPC Controllers/Path Following Controller ==
  Model : Inport
  mpc_mo_Vx : Inport  Port=2
  mpc_mo_e1 : Inport  Port=3
  mpc_mo_e2 : Inport  Port=4
  mpc_ref : Inport  Port=5
  mpc_md : Inport  Port=6
  mpc_ext_mv : Inport  Port=7
  mpc_umin : Inport  Port=8
  mpc_umax : Inport  Port=9
  mpc_switch : Inport  Port=10
  Adaptive MPC Controller : mpclib/Adaptive MPC Controller  SCDEnableBlockLinearizationSpecification=on  mpcobj=mpcobj  enable_value=0  updateMPCinCallerWorkspace=off  md_inport=on  mv_inport=off  uref_inport=off  return_cost=off  return_mvseq=off  return_qpstatus=off  return_xseq=off  return_state=off  return_ovseq=off  state_inport=off  isltv_plant=off  umin_inport=on  umax_inport=on  ymin_inport=off  ymax_inport=off  cc_inport=off  ywt_inport=off  uwt_inport=off  duwt_inport=off  rhoeps_inport=off  pm_inport=off  MaximumP=10  HorizonChoice=FixedHorizon  BlockDataType=double  SampleTimeInherited=off  switch_inport=on
  Demux : Demux  Outputs=2
  Mux : Mux  Inputs=3
  Track mv terminator : Terminator
  Longitudinal acceleration : Outport  Unit=m/s^2  VectorParamsAs1DForOutWhenUnconnected=off
  " Steering angle" : Outport  Port=2  Unit=rad  VectorParamsAs1DForOutWhenUnconnected=off
  wires:
  mpc_mo_Vx/1 -> Mux/1
  Adaptive MPC Controller/1 -> Demux/1
  Mux/1 -> Adaptive MPC Controller/2
  Model/1 -> Adaptive MPC Controller/1
  mpc_mo_e2/1 -> Mux/3
  mpc_mo_e1/1 -> Mux/2
  mpc_ref/1 -> Adaptive MPC Controller/3
  mpc_md/1 -> Adaptive MPC Controller/4
  mpc_umax/1 -> Adaptive MPC Controller/6
  mpc_umin/1 -> Adaptive MPC Controller/5
  mpc_switch/1 -> Adaptive MPC Controller/7
  Demux/1 -> Longitudinal acceleration/1
  Demux/2 -> " Steering angle"/1
  mpc_ext_mv/1 -> Track mv terminator/1

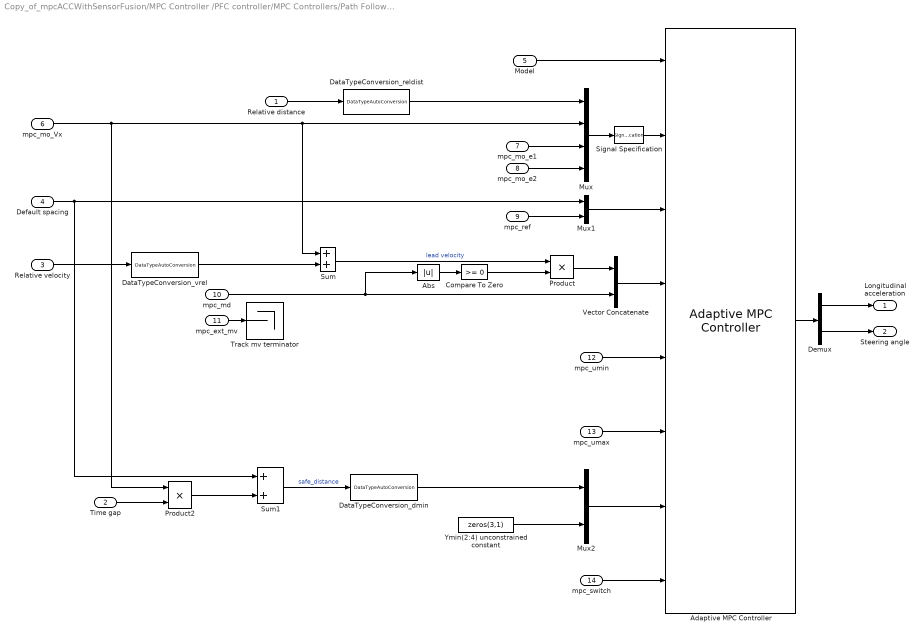
== system Copy_of_mpcACCWithSensorFusion/MPC Controller /PFC controller/MPC Controllers/Path Following Controller with Spacing Control ==
  Relative distance : Inport  Unit=m
  Time gap : Inport  Port=2
  Relative velocity : Inport  Port=3  Unit=m/s
  Default spacing : Inport  Port=4
  Model : Inport  Port=5
  mpc_mo_Vx : Inport  Port=6
  mpc_mo_e1 : Inport  Port=7
  mpc_mo_e2 : Inport  Port=8
  mpc_ref : Inport  Port=9
  mpc_md : Inport  Port=10
  mpc_ext_mv : Inport  Port=11
  mpc_umin : Inport  Port=12
  mpc_umax : Inport  Port=13
  mpc_switch : Inport  Port=14
  Abs : Abs  ZeroCross=off  SaturateOnIntegerOverflow=off
  Adaptive MPC Controller : mpclib/Adaptive MPC Controller  SCDEnableBlockLinearizationSpecification=on  mpcobj=pfcsubsystem_data.Controller  enable_value=0  updateMPCinCallerWorkspace=off  md_inport=on  mv_inport=off  uref_inport=off  return_cost=off  return_mvseq=off  return_qpstatus=off  return_xseq=off  return_state=off  return_ovseq=off  state_inport=off  isltv_plant=off  umin_inport=on  umax_inport=on  ymin_inport=on  ymax_inport=off  cc_inport=off  ywt_inport=off  uwt_inport=off  duwt_inport=off  rhoeps_inport=off  pm_inport=off  MaximumP=10  HorizonChoice=FixedHorizon  BlockDataType=double  SampleTimeInherited=off  switch_inport=on
  Compare To Zero : simulink/Logic and Bit Operations/Compare To Zero  relop=>=  OutDataTypeStr=boolean  ZeroCross=off
  DataTypeConversion_dmin : mpcsigdimcheck_private/DataTypeAutoConversion  datatypestr=pfcsubsystem_data.DataType
  DataTypeConversion_reldist : mpcsigdimcheck_private/DataTypeAutoConversion  datatypestr=pfcsubsystem_data.DataType
  DataTypeConversion_vrel : mpcsigdimcheck_private/DataTypeAutoConversion  datatypestr=pfcsubsystem_data.DataType
  Demux : Demux  Outputs=2
  Mux : Mux
  Mux1 : Mux  Inputs=2
  Mux2 : Mux  Inputs=2
  Product : Product
  Product2 : Product
  Signal Specification : SignalSpecification  Dimensions=4
  Sum : Sum
  Sum1 : Sum
  Track mv terminator : Terminator
  Vector Concatenate : Concatenate  Mode=Multidimensional array  ConcatenateDimension=2
  Ymin(2:4) unconstrained constant : Constant  Value=zeros(3,1)  VectorParams1D=off  OutDataTypeStr=pfcsubsystem_data.DataType
  Longitudinal acceleration : Outport  Unit=m/s^2  VectorParamsAs1DForOutWhenUnconnected=off
  " Steering angle" : Outport  Port=2  Unit=rad  VectorParamsAs1DForOutWhenUnconnected=off
  wires:
  Mux2/1 -> Adaptive MPC Controller/7
  Ymin(2:4) unconstrained constant/1 -> Mux2/2
  DataTypeConversion_reldist/1 -> Mux/1
  mpc_umin/1 -> Adaptive MPC Controller/5
  Demux/1 -> Longitudinal acceleration/1
  Model/1 -> Adaptive MPC Controller/1
  mpc_mo_e2/1 -> Mux/4
  Mux/1 -> Signal Specification/1
  Default spacing/1 -> Mux1/1, Sum1/1
  Relative velocity/1 -> DataTypeConversion_vrel/1
  mpc_mo_Vx/1 -> Product2/1, Mux/2, Sum/1
  mpc_umax/1 -> Adaptive MPC Controller/6
  Mux1/1 -> Adaptive MPC Controller/3
  Relative distance/1 -> DataTypeConversion_reldist/1
  Product2/1 -> Sum1/2
  mpc_switch/1 -> Adaptive MPC Controller/8
  Adaptive MPC Controller/1 -> Demux/1
  mpc_mo_e1/1 -> Mux/3
  Time gap/1 -> Product2/2
  Sum1/1 -> DataTypeConversion_dmin/1  "safe_distance"
  Sum/1 -> Product/1  "lead velocity"
  Demux/2 -> " Steering angle"/1
  DataTypeConversion_dmin/1 -> Mux2/1
  Signal Specification/1 -> Adaptive MPC Controller/2
  Vector Concatenate/1 -> Adaptive MPC Controller/4
  mpc_ref/1 -> Mux1/2
  mpc_ext_mv/1 -> Track mv terminator/1
  DataTypeConversion_vrel/1 -> Sum/2
  Abs/1 -> Compare To Zero/1
  mpc_md/1 -> Abs/1, Vector Concatenate/2
  Compare To Zero/1 -> Product/2
  Product/1 -> Vector Concatenate/1

== system Copy_of_mpcACCWithSensorFusion/MPC Controller /PFC controller/MPC Models/MPC Model ==
  Sample time : Inport
  Transport lag : Inport  Port=2
  Longitudinal velocity : Inport  Port=3
  Ag : Inport  Port=4
  Bg : Inport  Port=5
  Cg : Inport  Port=6
  Adaptive Model : MATLAB Function  TreatAsAtomicUnit=on
  Bus Creator2 : BusCreator  Inputs=8
  DX Constant : Constant  Value=zeros(NumEgoStates+2+3*hasLag,1)  VectorParams1D=off  OutDataTypeStr=pfcsubsystem_data.DataType
  U Constant : Constant  Value=zeros(3,1)  VectorParams1D=off  OutDataTypeStr=pfcsubsystem_data.DataType
  X Constant : Constant  Value=zeros(NumEgoStates+2+3*hasLag,1)  VectorParams1D=off  OutDataTypeStr=pfcsubsystem_data.DataType
  Y Constant : Constant  Value=[InitialLongVel;0;0]  VectorParams1D=off  OutDataTypeStr=pfcsubsystem_data.DataType
  Model : Outport  VectorParamsAs1DForOutWhenUnconnected=off
  wires:
  Adaptive Model/2(B) -> Bus Creator2/2  "B"
  Transport lag/1 -> Adaptive Model/6(lag)
  U Constant/1 -> Bus Creator2/5  "U"
  DX Constant/1 -> Bus Creator2/8  "DX"
  Adaptive Model/3(C) -> Bus Creator2/3  "C"
  Adaptive Model/4(D) -> Bus Creator2/4  "D"
  Longitudinal velocity/1 -> Adaptive Model/2(Vx)
  Adaptive Model/1(A) -> Bus Creator2/1  "A"
  Sample time/1 -> Adaptive Model/1(Ts)
  Y Constant/1 -> Bus Creator2/6  "Y"
  X Constant/1 -> Bus Creator2/7  "X"
  Bus Creator2/1 -> Model/1
  Ag/1 -> Adaptive Model/3(Ag)
  Bg/1 -> Adaptive Model/4(Bg)
  Cg/1 -> Adaptive Model/5(Cg)

== system Copy_of_mpcACCWithSensorFusion/MPC Controller /PFC controller/MPC Models/MPC Model with Spacing Control ==
  Sample time : Inport
  Transport lag : Inport  Port=2
  Longitudinal velocity : Inport  Port=3
  Ag : Inport  Port=4
  Bg : Inport  Port=5
  Cg : Inport  Port=6
  Adaptive Model with Spacing Control : MATLAB Function  TreatAsAtomicUnit=on
  Bus Creator2 : BusCreator  Inputs=8
  DX Constant : Constant  Value=zeros(pfcsubsystem_data.NumEgoStates+3+4*pfcsubsystem_data.hasLag,1)  VectorParams1D=off  OutDataTypeStr=pfcsubsystem_data.DataType
  U Constant : Constant  Value=[0;0;pfcsubsystem_data.InitialLongVel;0]  VectorParams1D=off  OutDataTypeStr=pfcsubsystem_data.DataType
  X Constant : Constant  Value=zeros(pfcsubsystem_data.NumEgoStates+3+4*pfcsubsystem_data.hasLag,1)  VectorParams1D=off  OutDataTypeStr=pfcsubsystem_data.DataType
  Y Constant : Constant  Value=[1.4*pfcsubsystem_data.InitialLongVel+pfcsubsystem_data.DefaultSpacing;pfcsubsystem_data.InitialLongVel;0;0]  VectorParams1D=off  OutDataTypeStr=pfcsubsystem_data.DataType
  Model : Outport  VectorParamsAs1DForOutWhenUnconnected=off
  wires:
  Adaptive Model with Spacing Control/4(D) -> Bus Creator2/4  "D"
  X Constant/1 -> Bus Creator2/7  "X"
  Bus Creator2/1 -> Model/1
  Sample time/1 -> Adaptive Model with Spacing Control/1(Ts)
  Adaptive Model with Spacing Control/1(A) -> Bus Creator2/1  "A"
  DX Constant/1 -> Bus Creator2/8  "DX"
  Adaptive Model with Spacing Control/2(B) -> Bus Creator2/2  "B"
  Adaptive Model with Spacing Control/3(C) -> Bus Creator2/3  "C"
  Longitudinal velocity/1 -> Adaptive Model with Spacing Control/2(Vx)
  Y Constant/1 -> Bus Creator2/6  "Y"
  U Constant/1 -> Bus Creator2/5  "U"
  Ag/1 -> Adaptive Model with Spacing Control/3(Ag)
  Bg/1 -> Adaptive Model with Spacing Control/4(Bg)
  Cg/1 -> Adaptive Model with Spacing Control/5(Cg)
  Transport lag/1 -> Adaptive Model with Spacing Control/6(lag)

== system Copy_of_mpcACCWithSensorFusion/MPC Controller /PFC controller/Vehicle Models/Vehicle external model ==
  Vehicle dynamics matrix A : Inport
  Vehicle dynamics matrix B : Inport  Port=2
  Vehicle dynamics matrix C : Inport  Port=3
  DataTypeConversion_A : mpcsigdimcheck_private/DataTypeAutoConversion2D  datatypestr=pfcsubsystem_data.DataType
  DataTypeConversion_B : mpcsigdimcheck_private/DataTypeAutoConversion2D  datatypestr=pfcsubsystem_data.DataType
  DataTypeConversion_C : mpcsigdimcheck_private/DataTypeAutoConversion2D  datatypestr=pfcsubsystem_data.DataType
  Signal Specification A : SignalSpecification
  Signal Specification B : SignalSpecification
  Signal Specification C : SignalSpecification
  A : Outport  VectorParamsAs1DForOutWhenUnconnected=off
  B : Outport  Port=2  VectorParamsAs1DForOutWhenUnconnected=off
  C : Outport  Port=3  VectorParamsAs1DForOutWhenUnconnected=off
  wires:
  Signal Specification B/1 -> B/1
  Signal Specification C/1 -> C/1
  DataTypeConversion_C/1 -> Signal Specification C/1
  Signal Specification A/1 -> A/1
  Vehicle dynamics matrix A/1 -> DataTypeConversion_A/1
  Vehicle dynamics matrix C/1 -> DataTypeConversion_C/1
  DataTypeConversion_A/1 -> Signal Specification A/1
  Vehicle dynamics matrix B/1 -> DataTypeConversion_B/1
  DataTypeConversion_B/1 -> Signal Specification B/1

== system Copy_of_mpcACCWithSensorFusion/MPC Controller /PFC controller/Vehicle Models/Vehicle parametric model ==
  Vx : Inport
  Vehicle combined dynamics : Subsystem
  Vehicle lateral dynamics : Subsystem
  Vehicle longitudinal dynamics : Subsystem
  A : Outport  VectorParamsAs1DForOutWhenUnconnected=off
  B : Outport  Port=2  VectorParamsAs1DForOutWhenUnconnected=off
  C : Outport  Port=3  VectorParamsAs1DForOutWhenUnconnected=off
  wires:
  Vehicle combined dynamics/3(C) -> C/1
  Vehicle combined dynamics/1(A) -> A/1
  Vehicle combined dynamics/2(B) -> B/1
  Vehicle lateral dynamics/1(Am) -> Vehicle combined dynamics/4(A2)
  Vehicle lateral dynamics/2(Bm) -> Vehicle combined dynamics/5(B2)
  Vehicle lateral dynamics/3(Cm) -> Vehicle combined dynamics/6(C2)
  Vehicle longitudinal dynamics/1(An) -> Vehicle combined dynamics/1(A1)
  Vehicle longitudinal dynamics/2(Bn) -> Vehicle combined dynamics/2(B1)
  Vehicle longitudinal dynamics/3(Cn) -> Vehicle combined dynamics/3(C1)
  Vx/1 -> Vehicle lateral dynamics/1(Vx)

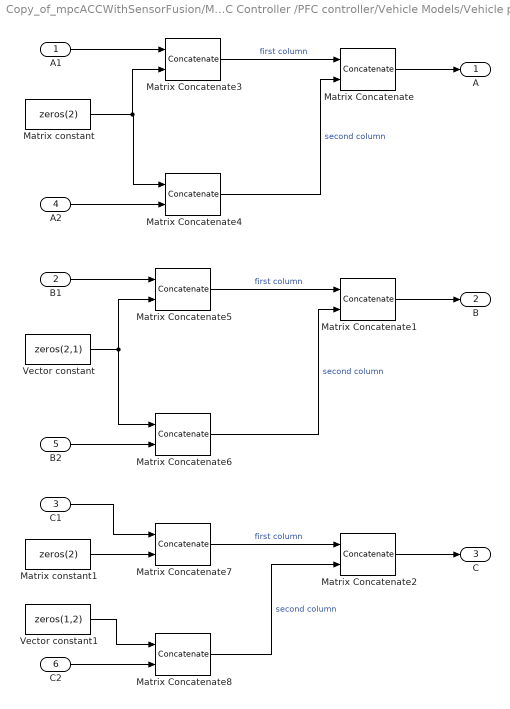
== system Copy_of_mpcACCWithSensorFusion/MPC Controller /PFC controller/Vehicle Models/Vehicle parametric model/Vehicle combined dynamics ==
  A1 : Inport
  B1 : Inport  Port=2
  C1 : Inport  Port=3
  A2 : Inport  Port=4
  B2 : Inport  Port=5
  C2 : Inport  Port=6
  Matrix Concatenate : Concatenate  Mode=Multidimensional array  ConcatenateDimension=2
  Matrix Concatenate1 : Concatenate  Mode=Multidimensional array  ConcatenateDimension=2
  Matrix Concatenate2 : Concatenate  Mode=Multidimensional array  ConcatenateDimension=2
  Matrix Concatenate{3..8} (6 alike) : Concatenate  Mode=Multidimensional array
  Matrix constant : Constant  Value=zeros(2)  VectorParams1D=off  OutDataTypeStr=pfcsubsystem_data.DataType
  Matrix constant1 : Constant  Value=zeros(2)  VectorParams1D=off  OutDataTypeStr=pfcsubsystem_data.DataType
  Vector constant : Constant  Value=zeros(2,1)  VectorParams1D=off  OutDataTypeStr=pfcsubsystem_data.DataType
  Vector constant1 : Constant  Value=zeros(1,2)  VectorParams1D=off  OutDataTypeStr=pfcsubsystem_data.DataType
  A : Outport  VectorParamsAs1DForOutWhenUnconnected=off
  B : Outport  Port=2  VectorParamsAs1DForOutWhenUnconnected=off
  C : Outport  Port=3  VectorParamsAs1DForOutWhenUnconnected=off
  wires:
  Vector constant/1 -> Matrix Concatenate6/1, Matrix Concatenate5/2
  C1/1 -> Matrix Concatenate7/1
  Matrix Concatenate6/1 -> Matrix Concatenate1/2  "second column"
  Matrix Concatenate4/1 -> Matrix Concatenate/2  "second column"
  B1/1 -> Matrix Concatenate5/1
  Matrix Concatenate1/1 -> B/1
  Vector constant1/1 -> Matrix Concatenate8/1
  Matrix Concatenate/1 -> A/1
  Matrix constant/1 -> Matrix Concatenate4/1, Matrix Concatenate3/2
  Matrix Concatenate2/1 -> C/1
  Matrix constant1/1 -> Matrix Concatenate7/2
  Matrix Concatenate8/1 -> Matrix Concatenate2/2  "second column"
  Matrix Concatenate7/1 -> Matrix Concatenate2/1  "first column"
  C2/1 -> Matrix Concatenate8/2
  B2/1 -> Matrix Concatenate6/2
  A2/1 -> Matrix Concatenate4/2
  Matrix Concatenate3/1 -> Matrix Concatenate/1  "first column"
  A1/1 -> Matrix Concatenate3/1
  Matrix Concatenate5/1 -> Matrix Concatenate1/1  "first column"

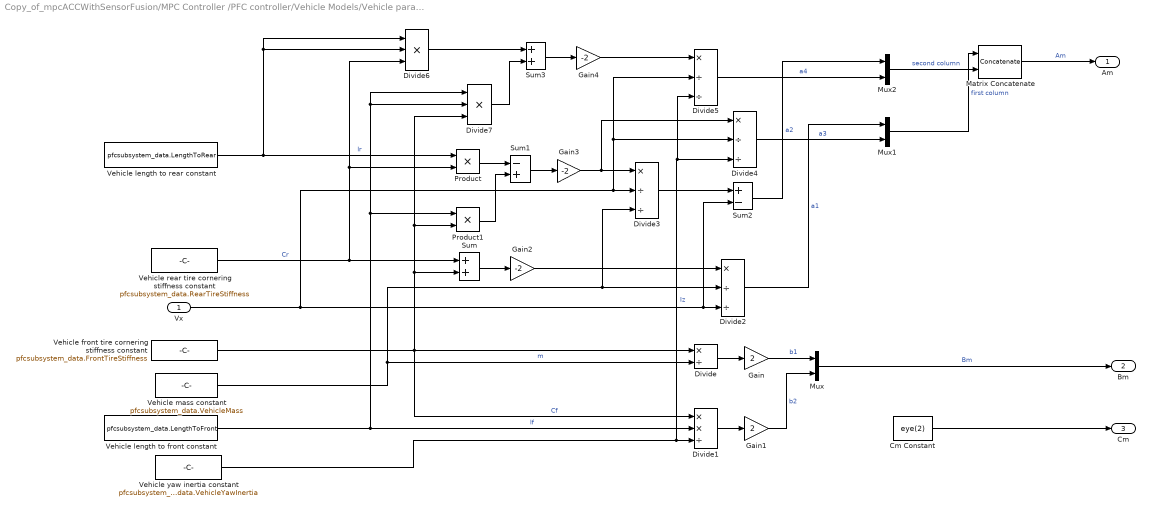
== system Copy_of_mpcACCWithSensorFusion/MPC Controller /PFC controller/Vehicle Models/Vehicle parametric model/Vehicle lateral dynamics ==
  Vx : Inport
  Cm Constant : Constant  Value=eye(2)  OutDataTypeStr=pfcsubsystem_data.DataType
  Divide : Product  Inputs=*/
  Divide1 : Product  Inputs=**/
  Divide{2..5} (4 alike) : Product  Inputs=*//
  Divide6 : Product  Inputs=***
  Divide7 : Product  Inputs=***
  Gain : Gain  Gain=2
  Gain1 : Gain  Gain=2
  Gain2 : Gain  Gain=-2
  Gain3 : Gain  Gain=-2
  Gain4 : Gain  Gain=-2
  Matrix Concatenate : Concatenate  Mode=Multidimensional array  ConcatenateDimension=2
  Mux : Mux  Inputs=[1 1]
  Mux1 : Mux  Inputs=[1 1]
  Mux2 : Mux  Inputs=[1 1]
  Product : Product
  Product1 : Product
  Sum : Sum
  Sum1 : Sum  Inputs=-+
  Sum2 : Sum  Inputs=+-
  Sum3 : Sum
  Vehicle front tire cornering stiffness constant : Constant  Value=pfcsubsystem_data.FrontTireStiffness  OutDataTypeStr=pfcsubsystem_data.DataType
  Vehicle length to front constant : Constant  Value=pfcsubsystem_data.LengthToFront  OutDataTypeStr=pfcsubsystem_data.DataType
  Vehicle length to rear constant : Constant  Value=pfcsubsystem_data.LengthToRear  OutDataTypeStr=pfcsubsystem_data.DataType
  Vehicle mass constant : Constant  Value=pfcsubsystem_data.VehicleMass  OutDataTypeStr=pfcsubsystem_data.DataType
  Vehicle rear tire cornering stiffness constant : Constant  Value=pfcsubsystem_data.RearTireStiffness  OutDataTypeStr=pfcsubsystem_data.DataType
  Vehicle yaw inertia constant : Constant  Value=pfcsubsystem_data.VehicleYawInertia  OutDataTypeStr=pfcsubsystem_data.DataType
  Am : Outport  VectorParamsAs1DForOutWhenUnconnected=off
  Bm : Outport  Port=2  VectorParamsAs1DForOutWhenUnconnected=off
  Cm : Outport  Port=3  VectorParamsAs1DForOutWhenUnconnected=off
  wires:
  Divide5/1 -> Mux2/2  "a4"
  Vehicle length to front constant/1 -> Divide7/1, Divide7/2, Product1/1, Divide1/2  "lf"
  Mux2/1 -> Matrix Concatenate/2  "second column"
  Product1/1 -> Sum1/2
  Vehicle front tire cornering stiffness constant/1 -> Divide1/1, Divide/1, Divide7/3, Product1/2, Sum/2  "Cf"
  Vehicle yaw inertia constant/1 -> Divide5/3, Divide4/3, Divide1/3  "Iz"
  Vehicle mass constant/1 -> Divide/2, Divide3/3, Divide2/2  "m"
  Gain4/1 -> Divide5/1
  Vehicle length to rear constant/1 -> Divide6/2, Divide6/1, Product/1  "lr"
  Vehicle rear tire cornering stiffness constant/1 -> Divide6/3, Product/2, Sum/1  "Cr"
  Sum2/1 -> Mux2/1  "a2"
  Vx/1 -> Divide3/2, Divide5/2, Divide4/2, Sum2/2, Divide2/3
  Gain/1 -> Mux/1  "b1"
  Divide2/1 -> Mux1/1  "a1"
  Product/1 -> Sum1/1
  Mux/1 -> Bm/1  "Bm"
  Divide4/1 -> Mux1/2  "a3"
  Divide7/1 -> Sum3/2
  Matrix Concatenate/1 -> Am/1  "Am"
  Sum3/1 -> Gain4/1
  Gain3/1 -> Divide3/1, Divide4/1
  Sum1/1 -> Gain3/1
  Mux1/1 -> Matrix Concatenate/1  "first column"
  Sum/1 -> Gain2/1
  Divide3/1 -> Sum2/1
  Gain1/1 -> Mux/2  "b2"
  Divide/1 -> Gain/1
  Divide1/1 -> Gain1/1
  Cm Constant/1 -> Cm/1
  Gain2/1 -> Divide2/1
  Divide6/1 -> Sum3/1

== system Copy_of_mpcACCWithSensorFusion/MPC Controller /PFC controller/Vehicle Models/Vehicle parametric model/Vehicle longitudinal dynamics ==
  Cn constant : Constant  Value=[0,1]  VectorParams1D=off  OutDataTypeStr=pfcsubsystem_data.DataType
  Divide : Product  Inputs=*/
  Matrix Concatenate : Concatenate  Mode=Multidimensional array  ConcatenateDimension=2
  Mux1 : Mux  Inputs=[1 1]
  Mux2 : Mux  Inputs=[1 1]
  Scalar one constant : Constant  OutDataTypeStr=pfcsubsystem_data.DataType
  Scalar zero constant : Constant  Value=0  OutDataTypeStr=pfcsubsystem_data.DataType
  Unary Minus : UnaryMinus
  Vector constant : Constant  Value=zeros(2,1)  VectorParams1D=off  OutDataTypeStr=pfcsubsystem_data.DataType
  Vehicle acceleration tracking time constant : Constant  Value=pfcsubsystem_data.AccelTimeConstant  OutDataTypeStr=pfcsubsystem_data.DataType
  An : Outport  VectorParamsAs1DForOutWhenUnconnected=off
  Bn : Outport  Port=2  VectorParamsAs1DForOutWhenUnconnected=off
  Cn : Outport  Port=3  VectorParamsAs1DForOutWhenUnconnected=off
  wires:
  Vehicle acceleration tracking time constant/1 -> Divide/2  "tau"
  Divide/1 -> Mux2/1, Unary Minus/1  "1/tau"
  Vector constant/1 -> Matrix Concatenate/2  "second column"
  Matrix Concatenate/1 -> An/1  "An"
  Cn constant/1 -> Cn/1  "Cn"
  Unary Minus/1 -> Mux1/1  "a1"
  Scalar one constant/1 -> Mux1/2, Divide/1  "a3"
  Mux2/1 -> Bn/1  "Bn"
  Scalar zero constant/1 -> Mux2/2
  Mux1/1 -> Matrix Concatenate/1  "first column"

== matlab function Copy_of_mpcACCWithSensorFusion/MPC Controller /PFC controller/MPC Models/MPC Model/Adaptive Model ==
  data: Ts input; A output; Vx input; Ag input; Bg input; Cg input; lag input; B output; C output; D output
function [A,B,C,D] = getAdaptiveMPCModel(Ts,Vx, Ag, Bg, Cg, lag)
% Get discrete state-space model for Adaptive MPC with sample time Ts.
% Called by the 'Path Following Control System' Block.

% Inputs:
%   Ts:               mask variable for sample time
%   Vx:               mask inport for longitudinal velocity
%   Ag,Bg,Cg:         continuous or discrete vehicle model with sample time Ts
% Outputs:
%   A,B,C,D:          discrete time model for adaptive MPC

%   Author: Meng Xia, Rong Chen
%   Copyright 2017-2018 The MathWorks, Inc.

% Discrete MPC model
[A,B,C,D] = pfcblock_utilGetDTModelHasLagForMPCNoSpacingCtrl(Ts,Vx,Ag,Bg,Cg,lag);
